simulink model "forward_converter_with_RCsnubber"  (R2018a)
settings: Solver=VariableStepAuto  StartTime=0.0  StopTime=0.1  FixedStep=1e-08  RelTol=1e-3
libraries: powerlib x22, pePowerMeasurement x3
settings Model: Creator=gizemlikaradenizli61  LastModifiedBy=anılcanbudak
settings SolverCC: AlgebraicLoopSolver=LineSearch

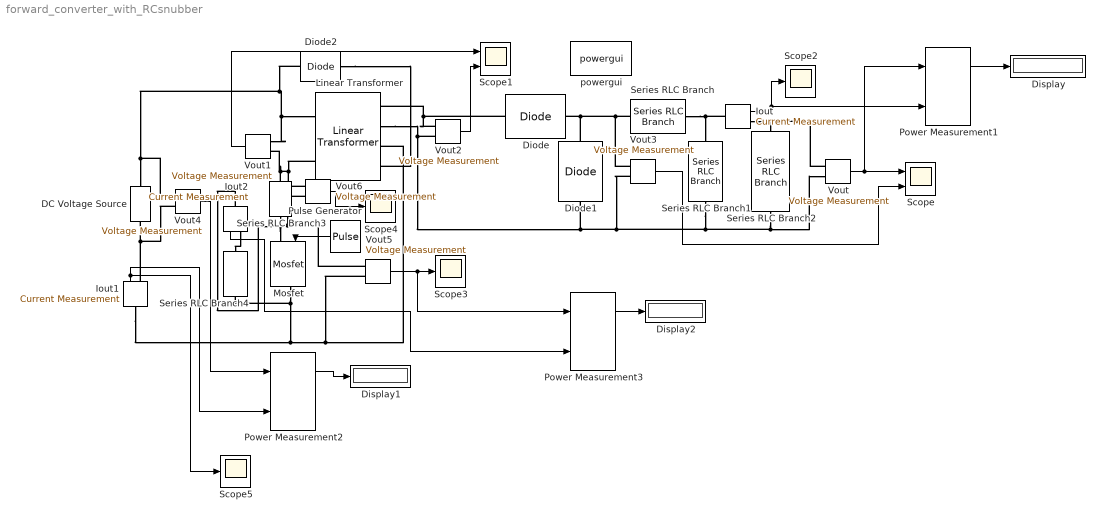
== system forward_converter_with_RCsnubber ==
  DC Voltage Source : powerlib/Electrical Sources/DC Voltage Source  Amplitude=48  Measurements=None
  Diode : powerlib/Power Electronics/Diode  Ron=0.0124  Lon=0  Vf=0.73  IC=0  UseSnubber=0  Rs=inf  Cs=inf  Measurements=off
  Diode1 : powerlib/Power Electronics/Diode  Ron=0.0124  Lon=0  Vf=0.73  IC=0  UseSnubber=0  Rs=inf  Cs=inf  Measurements=off
  Diode2 : powerlib/Power Electronics/Diode  Ron=0.0124  Lon=0  Vf=0.8  IC=0  UseSnubber=0  Rs=inf  Cs=inf  Measurements=off
  Display : Display
  Display1 : Display
  Display2 : Display
  Iout : powerlib/Measurements/Current Measurement  PhasorSimulation=off  OutputType=Complex  PSBequivalent=0
  Iout1 : powerlib/Measurements/Current Measurement  PhasorSimulation=off  OutputType=Complex  PSBequivalent=0
  Iout2 : powerlib/Measurements/Current Measurement  PhasorSimulation=off  OutputType=Complex  PSBequivalent=0
  Linear Transformer : powerlib/Elements/Linear Transformer  UNITS=SI  NominalPower=[ 40 30000]  winding1=[26 0.11 0]  winding2=[24 0.1 0]  ThreeWindings=on  winding3="[26 0.01  0]"  RmLm=[1e6 0]  Measurements=None  DataType=on
  Mosfet : powerlib/Power Electronics/Mosfet  Ron=0.9  Lon=0  Rd=0  Vfd=0.9  IC=0  Rs=inf  Cs=inf  Measurements=off
  Power Measurement1 : pePowerMeasurement/Power Measurement  OverrideUsingVariant=Discrete  F=30000  K=[0 1 2 3]  Ts=0.000001
  Power Measurement2 : pePowerMeasurement/Power Measurement  OverrideUsingVariant=Discrete  F=30000  K=[0 1 2 3]  Ts=0.000001
  Power Measurement3 : pePowerMeasurement/Power Measurement  OverrideUsingVariant=Discrete  F=30000  K=[0 1 2 3]  Ts=0.000001
  Pulse Generator : DiscretePulseGenerator  PulseType=Time based  Period=0.000033  PulseWidth=26.8
  Scope : Scope  NumInputPorts=2
  Scope1 : Scope  NumInputPorts=2
  Scope{2..5} (4 alike) : Scope
  Series RLC Branch : powerlib/Elements/Series RLC Branch  LConnTagsString=__new0  RConnTagsString=__new0  BranchType=L  Resistance=1  Inductance=5e-4  SetiL0=off  InitialCurrent=0  Capacitance=1e-6  Setx0=off  InitialVoltage=0  Measurements=None
  Series RLC Branch1 : powerlib/Elements/Series RLC Branch  LConnTagsString=__new0  RConnTagsString=__new0  BranchType=C  Resistance=1  Inductance=1e-3  SetiL0=off  InitialCurrent=0  Capacitance=100e-6  Setx0=off  InitialVoltage=0  Measurements=None
  Series RLC Branch2 : powerlib/Elements/Series RLC Branch  LConnTagsString=__new0  RConnTagsString=__new0  BranchType=R  Resistance=2.5  Inductance=1e-3  SetiL0=off  InitialCurrent=0  Capacitance=1e-6  Setx0=off  InitialVoltage=0  Measurements=None
  Series RLC Branch3 : powerlib/Elements/Series RLC Branch  LConnTagsString=__new0  RConnTagsString=__new0  BranchType=L  Resistance=1  Inductance=1e-7  SetiL0=off  InitialCurrent=0  Capacitance=1e-6  Setx0=off  InitialVoltage=0  Measurements=None
  Series RLC Branch4 : powerlib/Elements/Series RLC Branch  LConnTagsString=__new0  RConnTagsString=__new0  BranchType=RC  Resistance=50  Inductance=1e-6  SetiL0=off  InitialCurrent=0  Capacitance=47e-9  Setx0=off  InitialVoltage=0  Measurements=None
  Vout{,1..6} (7 alike) : powerlib/Measurements/Voltage Measurement  PhasorSimulation=off  OutputType=Complex  PSBequivalent=0
  powergui : powerlib/powergui  Priority=1  SimulationMode=Continuous  SampleTime=1e-8  frequency=60  Iterations=50  frequencyindice=0  Pbase=100e6  ErrMax=1e-4  UnitsV=kV  UnitsW=MW  buscounter=0  FunctionMessages=off  echomessages=off  EnableUseOfTLC=off  CurrentSourceSwitches=off  DisableSnubberDevices=off  DisableRonSwitches=off  DisableVfSwitches=off  DisplayEquations=off  SolverType=Tustin/Backward Euler (TBE)  Interpol=off  ExternalGateDelay=off  methode=off  Ts=100  x0status=blocks  SPID=on  SwTol=0  HookPort=off  RestoreLinks=warning  ResistiveCurrentMeasurement=off  Frange=[0:2:500]  Ylog=off  Xlog=on  ShowGrid=off  save=off  variable=ZData  structure=0  ZoomFFT=off  StartTime=0.0  cycles=1  DisplayStyle=1  fundamental=60  FreqAxis=off  MaxFrequency=1000  frequencyindicesteady=1  RmsSteady=1  display=off
  wires:
  Pulse Generator/1 -> Mosfet/1
  Vout1/1 -> Scope1/1
  Vout2/1 -> Scope1/2
  Vout/1 -> Power Measurement1/1, Scope/1
  Vout3/1 -> Scope/2
  Iout/1 -> Power Measurement1/2, Scope2/1
  Power Measurement1/1 -> Display/1
  Vout4/1 -> Power Measurement2/1
  Iout1/1 -> Scope5/1, Power Measurement2/2
  Power Measurement2/1 -> Display1/1
  Vout5/1 -> Power Measurement3/1, Scope3/1
  Vout6/1 -> Scope4/1
  Power Measurement3/1 -> Display2/1
  Iout2/1 -> Power Measurement3/2
  connections:
  Series RLC Branch2/RConn1 -- Vout/LConn2 -- Vout2/LConn2 -- Linear Transformer/RConn2 -- Diode1/LConn1 -- Vout3/LConn2 -- Series RLC Branch1/RConn1
  Diode1/RConn1 -- Series RLC Branch/LConn1 -- Vout3/LConn1 -- Diode/RConn1
  Iout/LConn1 -- Series RLC Branch/RConn1 -- Series RLC Branch1/LConn1
  Iout/RConn1 -- Vout/LConn1 -- Series RLC Branch2/LConn1
  Diode/LConn1 -- Vout2/LConn1 -- Linear Transformer/RConn1
  Iout1/LConn1 -- Series RLC Branch4/RConn1 -- Mosfet/RConn1 -- Vout5/LConn2 -- Linear Transformer/RConn3
  Vout1/LConn1 -- Diode2/RConn1 -- Vout4/LConn1 -- DC Voltage Source/RConn1 -- Linear Transformer/LConn1
  Vout4/LConn2 -- Iout1/RConn1 -- DC Voltage Source/LConn1
  Vout5/LConn1 -- Vout6/LConn2 -- Mosfet/LConn1 -- Iout2/LConn1 -- Series RLC Branch3/RConn1
  Linear Transformer/LConn2 -- Vout6/LConn1 -- Series RLC Branch3/LConn1 -- Vout1/LConn2
  Diode2/LConn1 -- Linear Transformer/RConn4
  Iout2/RConn1 -- Series RLC Branch4/LConn1
